simulink model "Robot_leg_1"  (R2017b)
settings: Solver=VariableStepAuto  StartTime=0.0  StopTime=10.0  RelTol=1e-3
model workspace: external: MATLAB File E:\Humanoid\Simscape model\Simscape_model_2\simscape_model\Robot_leg_2_DataFile.m (data not in the file)
values from neighbouring files (symbols this model uses):
  m = 0    [Trajectory_generation.m]    (also in Trajectory_generation_initial.m; final_gait.m)
  smiData =     [matlab_workspace.mat]
undefined symbols (not defined in the file or in its folder): X, Y, Z
libraries: sm_lib x64, simulink x61, nesl_utility x13
(part 1 of 2)
settings Model: Creator=Workstation-1  LastModifiedBy=Workstation-1
settings SolverCC: AlgebraicLoopSolver=LineSearch
settings DiagnosticsConfigSet: SimMechanicsRigidlyBoundBlock=none

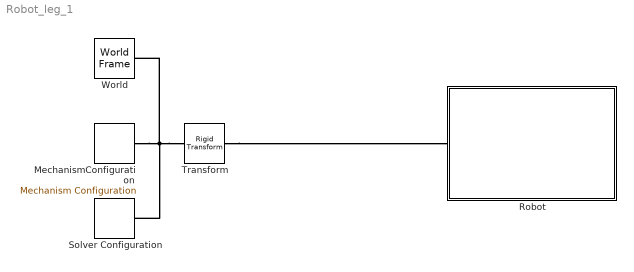
== system Robot_leg_1 ==
  MechanismConfiguration : sm_lib/Utilities/Mechanism Configuration  UniformGravity=Constant  GravityVector=[0 0 -9.80665]  GravityUnits=m/s^2  LinearizationDelta=0.001
  Robot : Subsystem
  Solver Configuration : nesl_utility/Solver Configuration  PhysicalDomain=network_engine_domain  SubClassName=solver  LeftPortType=input  RightPortType=generic  Accelerate=off  Tones=[]  Harmonics=[]  SimulateNoise=off  Profile=off  UseLocalSampling=off  EnableSwitchedLinearOptims=on  FrequencyDomain=off  UseCCode=off  RelTol=0.001  AbsTol=1e-06  MinStep=1e-09  ToWorkspace=off  RevertToSquareIcSolve=off  NumHomotopyIterations=100  PhasorMode=off  PhasorModeNumHarmonics=1  DoDC=off  ResidualTolerance=1e-09  UseLocalSolver=off  LocalSolverChoice=NE_BACKWARD_EULER_ADVANCER  LocalSolverSampleTime=0.001  DoFixedCost=off  MaxNonlinIter=3  MaxModeIter=2  LinearAlgebra=Sparse  DelaysMemoryBudget=1024  AutomaticFiltering=on  FilteringTimeConstant=0.001
  Transform : sm_lib/Frames and Transforms/Rigid Transform  TranslationMethod=Cartesian  TranslationStandardOffset=0  TranslationLengthUnit=mm  TranslationStandardAxis=+Z  TranslationCartesianOffset=smiData.RigidTransform(22).translation  TranslationROffset=0  TranslationROffsetUnits=m  TranslationZOffset=0  TranslationZOffsetUnits=m  TranslationThetaOffset=0  TranslationThetaOffsetUnits=deg  RotationMethod=ArbitraryAxis  RotationAngleUnits=rad  RotationStandardAxis=+Z  RotationAngle=smiData.RigidTransform(22).angle  RotationArbitraryAxis=smiData.RigidTransform(22).axis  FollAlignAxisA=+X  BaseAlignAxisA=+Y  FollAlignAxisB=+Y  BaseAlignAxisB=+Z  RotationSequenceAxes=FollowerAxes  RotationSequence=XYX  RotationSequenceAngles=[0 0 0]  RotationSequenceAnglesUnits=deg  RotationMatrix=[1 0 0; 0 1 0; 0 0 1]
  World : sm_lib/Frames and Transforms/World Frame
  connections:
  Transform/LConn1 -- Solver Configuration/RConn1 -- MechanismConfiguration/RConn1 -- World/RConn1
  Transform/RConn1 -- Robot/RConn1

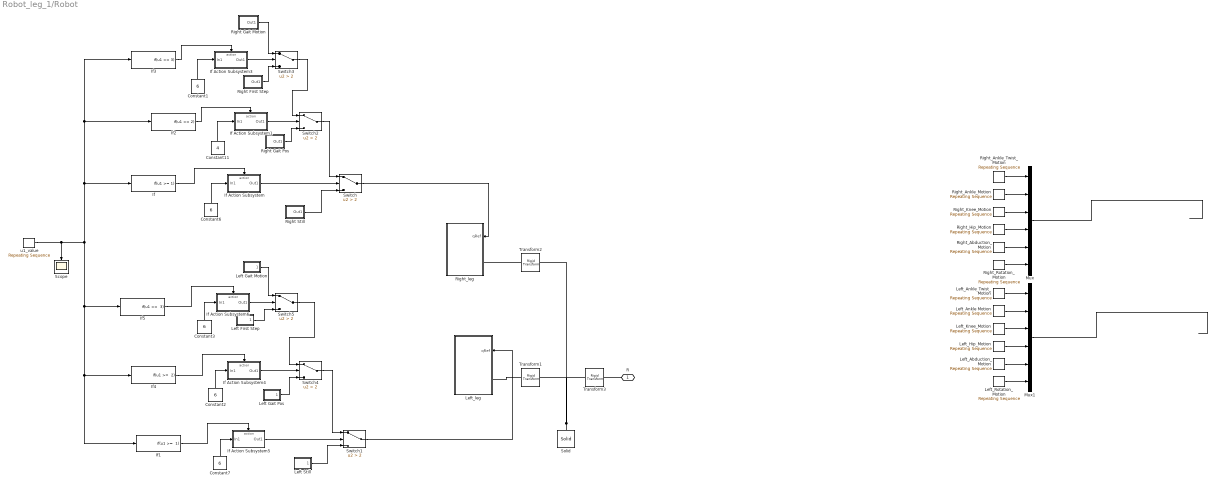
== system Robot_leg_1/Robot ==
  Constant{1..3,6..7} (5 alike) : Constant  Value=6
  Constant11 : Constant  Value=4
  If : If  IfExpression=u1 >= 1  ShowElse=off
  If Action Subsystem : Subsystem  TreatAsAtomicUnit=on
  If Action Subsystem1 : Subsystem  TreatAsAtomicUnit=on
  If Action Subsystem3 : Subsystem  TreatAsAtomicUnit=on
  If Action Subsystem4 : Subsystem  TreatAsAtomicUnit=on
  If Action Subsystem5 : Subsystem  TreatAsAtomicUnit=on
  If Action Subsystem6 : Subsystem  TreatAsAtomicUnit=on
  If1 : If  IfExpression="u1 >=  1"  ShowElse=off
  If2 : If  IfExpression=u1 >= 2  ShowElse=off
  If3 : If  IfExpression=u1 >= 3  ShowElse=off
  If4 : If  IfExpression="u1 >=  2"  ShowElse=off
  If5 : If  IfExpression="u1 >=  3"  ShowElse=off
  Left First Step : Subsystem
  Left Gait Motion : Subsystem
  Left Gait Pos : Subsystem
  Left Still : Subsystem
  Left_Abduction_Motion : simulink/Sources/Repeating Sequence  rep_seq_t=time  rep_seq_y=left_theta_5
  Left_Ankle Motion : simulink/Sources/Repeating Sequence  rep_seq_t=time  rep_seq_y=left_theta_3
  Left_Ankle_Twist_Motion : simulink/Sources/Repeating Sequence  rep_seq_t=time  rep_seq_y=left_theta_4
  Left_Hip_Motion : simulink/Sources/Repeating Sequence  rep_seq_t=time  rep_seq_y=left_theta_1
  Left_Knee_Motion : simulink/Sources/Repeating Sequence  rep_seq_t=time  rep_seq_y=left_theta_2
  Left_Rotation_Motion : simulink/Sources/Repeating Sequence  rep_seq_t=time  rep_seq_y=left_theta_6
  Left_leg : Subsystem
  Mux : Mux  Inputs=6
  Mux1 : Mux  Inputs=6
  Right First Step : Subsystem
  Right Gait Motion : Subsystem
  Right Gait Pos : Subsystem
  Right Still : Subsystem
  Right_Abduction_Motion : simulink/Sources/Repeating Sequence  rep_seq_t=time  rep_seq_y=right_theta_5
  Right_Ankle_Motion : simulink/Sources/Repeating Sequence  rep_seq_t=time  rep_seq_y=right_theta_3
  Right_Ankle_Twist_Motion : simulink/Sources/Repeating Sequence  rep_seq_t=time  rep_seq_y=right_theta_4
  Right_Hip_Motion : simulink/Sources/Repeating Sequence  rep_seq_t=time  rep_seq_y=right_theta_1
  Right_Knee_Motion : simulink/Sources/Repeating Sequence  rep_seq_t=time  rep_seq_y=right_theta_2
  Right_Rotation_Motion : simulink/Sources/Repeating Sequence  rep_seq_t=time  rep_seq_y=right_theta_6
  Right_leg : Subsystem
  Scope : Scope
  Solid : sm_lib/Body Elements/Solid  InertiaType=Custom  Mass=smiData.Solid(13).mass  MassUnits=kg  CenterOfMass=smiData.Solid(13).CoM  CenterOfMassUnits=mm  MomentsOfInertia=smiData.Solid(13).MoI  MomentsOfInertiaUnits=kg*mm^2  ProductsOfInertia=smiData.Solid(13).PoI  ProductsOfInertiaUnits=kg*mm^2  DensityBased=on  Density=1000  DensityUnits=kg/m^3  DoExposeReferenceFrame=on  SerializedFrames=<Frames/>  GraphicType=FromGeometry  MarkerShape=Sphere  MarkerSize=10  GraphicVisPropType=SimpleVisualProperties  GraphicDiffuseColor=smiData.Solid(13).color  GraphicSpecularColor=[0.5 0.5 0.5 1.0]  GraphicAmbientColor=[0.15 0.15 0.15 1.0]  GraphicEmissiveColor=[0.0 0.0 0.0 1.0]  GraphicShininess=75  GraphicOpacity=smiData.Solid(13).opacity  GeometryShape=FromFile  RectangleSize=[1 1]  RectangleSizeUnits=m  BrickDimensions=[1 1 1]  BrickDimensionUnits=m  CylinderRadius=1  CylinderRadiusUnits=m  CylinderLength=1  CylinderLengthUnits=m  SphereRadius=1  SphereRadiusUnits=m  EllipsoidRadii=[1 1 1]  EllipsoidRadiiUnits=m  ExtrusionCrossSection=[1 1; -1 1; -1 -1; 1 -1]  ExtrusionCrossSectionUnits=m  ExtrusionLength=1  ExtrusionLengthUnits=m  PolygonNumSides=3  PolygonOuterRadius=1  PolygonOuterRadiusUnits=m  ExtGeomFileType=STEP  ExtGeomFileName=Torso_Default_sldprt.STEP  ExtGeomFileUnits=m  RevolutionCrossSection=[1 1; 1 -1; 2 -1; 2 1]  RevolutionCrossSectionUnits=m  RevolutionExtent=Full  RevolutionAngle=180  RevolutionAngleUnits=deg
  Switch{,1..5} (6 alike) : Switch  Criteria=u2 > Threshold  Threshold=2
  Transform1 : sm_lib/Frames and Transforms/Rigid Transform  TranslationMethod=Cartesian  TranslationStandardOffset=0  TranslationLengthUnit=mm  TranslationStandardAxis=+Z  TranslationCartesianOffset=smiData.RigidTransform(17).translation  TranslationROffset=0  TranslationROffsetUnits=m  TranslationZOffset=0  TranslationZOffsetUnits=m  TranslationThetaOffset=0  TranslationThetaOffsetUnits=deg  RotationMethod=ArbitraryAxis  RotationAngleUnits=rad  RotationStandardAxis=+Z  RotationAngle=smiData.RigidTransform(17).angle  RotationArbitraryAxis=smiData.RigidTransform(17).axis  FollAlignAxisA=+X  BaseAlignAxisA=+Y  FollAlignAxisB=+Y  BaseAlignAxisB=+Z  RotationSequenceAxes=FollowerAxes  RotationSequence=XYX  RotationSequenceAngles=[0 0 0]  RotationSequenceAnglesUnits=deg  RotationMatrix=[1 0 0; 0 1 0; 0 0 1]
  Transform2 : sm_lib/Frames and Transforms/Rigid Transform  TranslationMethod=Cartesian  TranslationStandardOffset=0  TranslationLengthUnit=mm  TranslationStandardAxis=+Z  TranslationCartesianOffset=smiData.RigidTransform(19).translation  TranslationROffset=0  TranslationROffsetUnits=m  TranslationZOffset=0  TranslationZOffsetUnits=m  TranslationThetaOffset=0  TranslationThetaOffsetUnits=deg  RotationMethod=ArbitraryAxis  RotationAngleUnits=rad  RotationStandardAxis=+Z  RotationAngle=smiData.RigidTransform(19).angle  RotationArbitraryAxis=smiData.RigidTransform(19).axis  FollAlignAxisA=+X  BaseAlignAxisA=+Y  FollAlignAxisB=+Y  BaseAlignAxisB=+Z  RotationSequenceAxes=FollowerAxes  RotationSequence=XYX  RotationSequenceAngles=[0 0 0]  RotationSequenceAnglesUnits=deg  RotationMatrix=[1 0 0; 0 1 0; 0 0 1]
  Transform3 : sm_lib/Frames and Transforms/Rigid Transform  TranslationMethod=Cartesian  TranslationStandardOffset=0  TranslationLengthUnit=mm  TranslationStandardAxis=+Z  TranslationCartesianOffset=smiData.RigidTransform(21).translation  TranslationROffset=0  TranslationROffsetUnits=m  TranslationZOffset=0  TranslationZOffsetUnits=m  TranslationThetaOffset=0  TranslationThetaOffsetUnits=deg  RotationMethod=ArbitraryAxis  RotationAngleUnits=rad  RotationStandardAxis=+Z  RotationAngle=smiData.RigidTransform(21).angle  RotationArbitraryAxis=smiData.RigidTransform(21).axis  FollAlignAxisA=+X  BaseAlignAxisA=+Y  FollAlignAxisB=+Y  BaseAlignAxisB=+Z  RotationSequenceAxes=FollowerAxes  RotationSequence=XYX  RotationSequenceAngles=[0 0 0]  RotationSequenceAnglesUnits=deg  RotationMatrix=[1 0 0; 0 1 0; 0 0 1]
  "u1_value " : simulink/Sources/Repeating Sequence  rep_seq_t=total_time  rep_seq_y=u1
  R : PMIOPort  Port=1  Side=Right
  wires:
  If Action Subsystem1/1(Out1) -> Switch2/2
  If3/1 -> If Action Subsystem3/Action
  Constant3/1 -> If Action Subsystem6/1(In1)
  If5/1 -> If Action Subsystem6/Action
  Switch4/1 -> Switch1/1
  If Action Subsystem3/1(Out1) -> Switch3/2
  If4/1 -> If Action Subsystem4/Action
  Constant2/1 -> If Action Subsystem4/1(In1)
  If Action Subsystem5/1(Out1) -> Switch1/2
  If Action Subsystem6/1(Out1) -> Switch5/2
  Switch3/1 -> Switch2/1
  If Action Subsystem/1(Out1) -> Switch/2
  Constant7/1 -> If Action Subsystem5/1(In1)
  If/1 -> If Action Subsystem/Action
  If Action Subsystem4/1(Out1) -> Switch4/2
  Constant1/1 -> If Action Subsystem3/1(In1)
  If2/1 -> If Action Subsystem1/Action
  Switch5/1 -> Switch4/1
  Left Gait Pos/1(Out1) -> Switch4/3
  Constant6/1 -> If Action Subsystem/1(In1)
  Switch2/1 -> Switch/1
  If1/1 -> If Action Subsystem5/Action
  Constant11/1 -> If Action Subsystem1/1(In1)
  Left_Rotation_Motion/1 -> Mux1/6
  Left_Knee_Motion/1 -> Mux1/3
  Left_Hip_Motion/1 -> Mux1/4
  Left_Ankle_Twist_Motion/1 -> Mux1/1
  Right_Rotation_Motion/1 -> Mux/6
  Mux1/1 -> ?
  Right_Ankle_Motion/1 -> Mux/2
  Mux/1 -> ?
  Left_Abduction_Motion/1 -> Mux1/5
  Right_Abduction_Motion/1 -> Mux/5
  Right_Knee_Motion/1 -> Mux/3
  Right_Hip_Motion/1 -> Mux/4
  Left_Ankle Motion/1 -> Mux1/2
  Right_Ankle_Twist_Motion/1 -> Mux/1
  Switch/1 -> Right_leg/1(qRef)
  Switch1/1 -> Left_leg/1(qRef)
  Left First Step/1(Out1) -> Switch5/3
  Right Gait Pos/1(Out1) -> Switch2/3
  "u1_value "/1 -> Scope/1, If5/1, If4/1, If1/1, If2/1, If3/1, If/1
  Right First Step/1(Out1) -> Switch3/3
  Right Gait Motion/1(Out1) -> Switch3/1
  Right Still/1(Out1) -> Switch/3
  Left Gait Motion/1(Out1) -> Switch5/1
  Left Still/1(Out1) -> Switch1/3
  connections:
  Solid/RConn1 -- Transform2/LConn1 -- Transform1/LConn1 -- Transform3/LConn1
  R/RConn1 -- Transform3/RConn1
  Transform2/RConn1 -- Right_leg/LConn1
  Transform1/RConn1 -- Left_leg/LConn1

== system Robot_leg_1/Robot/If Action Subsystem ==
  In1 : Inport
  Action Port : ActionPort  ActionType=then
  Out1 : Outport
  wires:
  In1/1 -> Out1/1

== system Robot_leg_1/Robot/If Action Subsystem1 ==
  In1 : Inport
  Action Port : ActionPort  ActionType=then
  Out1 : Outport
  wires:
  In1/1 -> Out1/1

== system Robot_leg_1/Robot/If Action Subsystem3 ==
  In1 : Inport
  Action Port : ActionPort  ActionType=then
  Out1 : Outport
  wires:
  In1/1 -> Out1/1

== system Robot_leg_1/Robot/If Action Subsystem4 ==
  In1 : Inport
  Action Port : ActionPort  ActionType=then
  Out1 : Outport
  wires:
  In1/1 -> Out1/1

== system Robot_leg_1/Robot/If Action Subsystem5 ==
  In1 : Inport
  Action Port : ActionPort  ActionType=then
  Out1 : Outport
  wires:
  In1/1 -> Out1/1

== system Robot_leg_1/Robot/If Action Subsystem6 ==
  In1 : Inport
  Action Port : ActionPort  ActionType=then
  Out1 : Outport
  wires:
  In1/1 -> Out1/1

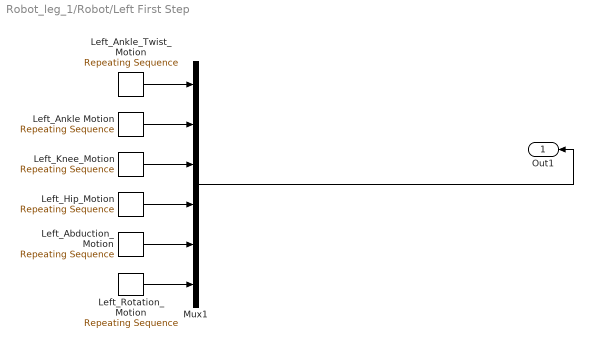
== system Robot_leg_1/Robot/Left First Step ==
  Left_Abduction_Motion : simulink/Sources/Repeating Sequence  rep_seq_t=time  rep_seq_y=left_theta_first_5
  Left_Ankle Motion : simulink/Sources/Repeating Sequence  rep_seq_t=time_first  rep_seq_y=left_theta_first_3
  Left_Ankle_Twist_Motion : simulink/Sources/Repeating Sequence  rep_seq_t=time  rep_seq_y=left_theta_first_4
  Left_Hip_Motion : simulink/Sources/Repeating Sequence  rep_seq_t=time_first  rep_seq_y=left_theta_first_1
  Left_Knee_Motion : simulink/Sources/Repeating Sequence  rep_seq_t=time_first  rep_seq_y=left_theta_first_2
  Left_Rotation_Motion : simulink/Sources/Repeating Sequence  rep_seq_t=time_first  rep_seq_y=left_theta_first_6
  Mux1 : Mux  Inputs=6
  Out1 : Outport
  wires:
  Left_Knee_Motion/1 -> Mux1/3
  Left_Rotation_Motion/1 -> Mux1/6
  Left_Hip_Motion/1 -> Mux1/4
  Left_Abduction_Motion/1 -> Mux1/5
  Left_Ankle_Twist_Motion/1 -> Mux1/1
  Left_Ankle Motion/1 -> Mux1/2
  Mux1/1 -> Out1/1

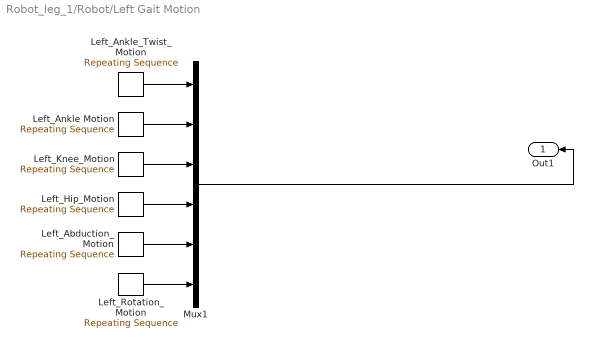
== system Robot_leg_1/Robot/Left Gait Motion ==
  Left_Abduction_Motion : simulink/Sources/Repeating Sequence  rep_seq_t=time  rep_seq_y=left_theta_5
  Left_Ankle Motion : simulink/Sources/Repeating Sequence  rep_seq_t=time  rep_seq_y=left_theta_3
  Left_Ankle_Twist_Motion : simulink/Sources/Repeating Sequence  rep_seq_t=time  rep_seq_y=left_theta_4
  Left_Hip_Motion : simulink/Sources/Repeating Sequence  rep_seq_t=time  rep_seq_y=left_theta_1
  Left_Knee_Motion : simulink/Sources/Repeating Sequence  rep_seq_t=time  rep_seq_y=left_theta_2
  Left_Rotation_Motion : simulink/Sources/Repeating Sequence  rep_seq_t=time  rep_seq_y=left_theta_6
  Mux1 : Mux  Inputs=6
  Out1 : Outport
  wires:
  Left_Knee_Motion/1 -> Mux1/3
  Left_Rotation_Motion/1 -> Mux1/6
  Left_Hip_Motion/1 -> Mux1/4
  Left_Abduction_Motion/1 -> Mux1/5
  Left_Ankle_Twist_Motion/1 -> Mux1/1
  Left_Ankle Motion/1 -> Mux1/2
  Mux1/1 -> Out1/1

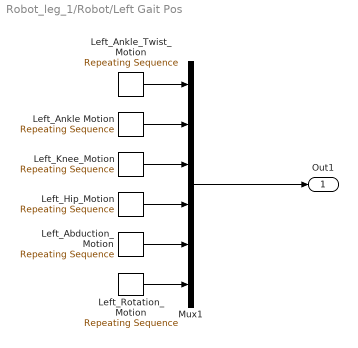
== system Robot_leg_1/Robot/Left Gait Pos ==
  Left_Abduction_Motion : simulink/Sources/Repeating Sequence  rep_seq_t=time  rep_seq_y=left_theta_pos_5
  Left_Ankle Motion : simulink/Sources/Repeating Sequence  rep_seq_t=time  rep_seq_y=left_theta_pos_3
  Left_Ankle_Twist_Motion : simulink/Sources/Repeating Sequence  rep_seq_t=time  rep_seq_y=left_theta_pos_4
  Left_Hip_Motion : simulink/Sources/Repeating Sequence  rep_seq_t=time  rep_seq_y=left_theta_pos_1
  Left_Knee_Motion : simulink/Sources/Repeating Sequence  rep_seq_t=time  rep_seq_y=left_theta_pos_2
  Left_Rotation_Motion : simulink/Sources/Repeating Sequence  rep_seq_t=time  rep_seq_y=left_theta_pos_6
  Mux1 : Mux  Inputs=6
  Out1 : Outport
  wires:
  Mux1/1 -> Out1/1
  Left_Ankle Motion/1 -> Mux1/2
  Left_Ankle_Twist_Motion/1 -> Mux1/1
  Left_Abduction_Motion/1 -> Mux1/5
  Left_Hip_Motion/1 -> Mux1/4
  Left_Rotation_Motion/1 -> Mux1/6
  Left_Knee_Motion/1 -> Mux1/3

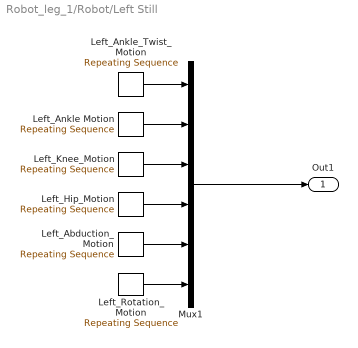
== system Robot_leg_1/Robot/Left Still ==
  Left_Abduction_Motion : simulink/Sources/Repeating Sequence  rep_seq_t=time  rep_seq_y=left_theta_init_5
  Left_Ankle Motion : simulink/Sources/Repeating Sequence  rep_seq_t=time  rep_seq_y=left_theta_init_3
  Left_Ankle_Twist_Motion : simulink/Sources/Repeating Sequence  rep_seq_t=time  rep_seq_y=left_theta_init_4
  Left_Hip_Motion : simulink/Sources/Repeating Sequence  rep_seq_t=time  rep_seq_y=left_theta_init_1
  Left_Knee_Motion : simulink/Sources/Repeating Sequence  rep_seq_t=time  rep_seq_y=left_theta_init_2
  Left_Rotation_Motion : simulink/Sources/Repeating Sequence  rep_seq_t=time  rep_seq_y=left_theta_init_6
  Mux1 : Mux  Inputs=6
  Out1 : Outport
  wires:
  Mux1/1 -> Out1/1
  Left_Ankle Motion/1 -> Mux1/2
  Left_Ankle_Twist_Motion/1 -> Mux1/1
  Left_Abduction_Motion/1 -> Mux1/5
  Left_Hip_Motion/1 -> Mux1/4
  Left_Rotation_Motion/1 -> Mux1/6
  Left_Knee_Motion/1 -> Mux1/3

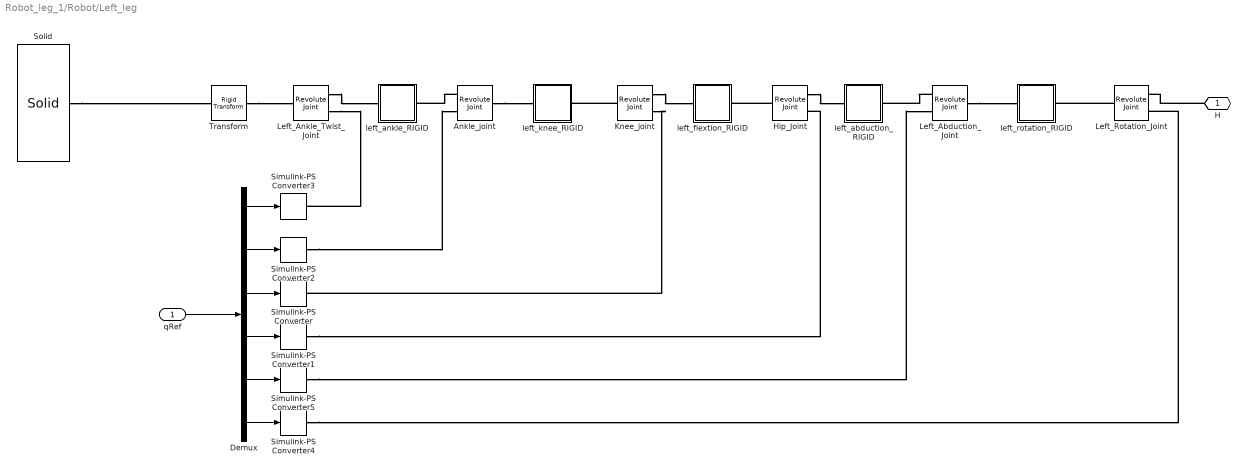
== system Robot_leg_1/Robot/Left_leg ==
  qRef : Inport
  Ankle_joint : sm_lib/Joints/Revolute Joint  SenseConstraintForce=off  SenseConstraintForceX=off  SenseConstraintForceY=off  SenseConstraintForceZ=off  SenseConstraintTorque=off  SenseConstraintTorqueX=off  SenseConstraintTorqueY=off  SenseConstraintTorqueZ=off  SenseTotalForce=off  SenseTotalForceX=off  SenseTotalForceY=off  SenseTotalForceZ=off  SenseTotalTorque=off  SenseTotalTorqueX=off  SenseTotalTorqueY=off  SenseTotalTorqueZ=off  CompositeWrenchDir=FollowerOnBase  CompositeWrenchFrame=BaseFrame  EquilibriumPosition=0  EquilibriumPositionUnits=rad  SpringStiffness=0  SpringStiffnessUnits=N*m/rad  DampingCoefficient=0  DampingCoefficientUnits=N*m/(rad/s)  TorqueActuationMode=ComputedTorque  MotionActuationMode=InputMotion  SensePosition=off  SenseVelocity=off  SenseAcceleration=off  SenseTorqueForce=off  PositionTargetSpecify=on  PositionTargetPriority=Low  PositionTargetValue=smiData.RevoluteJoint(7).Rz.Pos  PositionTargetValueUnits=deg  VelocityTargetSpecify=off  VelocityTargetPriority=High  VelocityTargetValue=0  VelocityTargetValueUnits=deg/s
  Demux : Demux  Outputs=6
  Hip_Joint : sm_lib/Joints/Revolute Joint  SenseConstraintForce=off  SenseConstraintForceX=off  SenseConstraintForceY=off  SenseConstraintForceZ=off  SenseConstraintTorque=off  SenseConstraintTorqueX=off  SenseConstraintTorqueY=off  SenseConstraintTorqueZ=off  SenseTotalForce=off  SenseTotalForceX=off  SenseTotalForceY=off  SenseTotalForceZ=off  SenseTotalTorque=off  SenseTotalTorqueX=off  SenseTotalTorqueY=off  SenseTotalTorqueZ=off  CompositeWrenchDir=FollowerOnBase  CompositeWrenchFrame=BaseFrame  EquilibriumPosition=0  EquilibriumPositionUnits=rad  SpringStiffness=0  SpringStiffnessUnits=N*m/rad  DampingCoefficient=0  DampingCoefficientUnits=N*m/(rad/s)  TorqueActuationMode=ComputedTorque  MotionActuationMode=InputMotion  SensePosition=off  SenseVelocity=off  SenseAcceleration=off  SenseTorqueForce=off  PositionTargetSpecify=on  PositionTargetPriority=Low  PositionTargetValue=smiData.RevoluteJoint(12).Rz.Pos  PositionTargetValueUnits=deg  VelocityTargetSpecify=off  VelocityTargetPriority=High  VelocityTargetValue=0  VelocityTargetValueUnits=deg/s
  Knee_joint : sm_lib/Joints/Revolute Joint  SenseConstraintForce=off  SenseConstraintForceX=off  SenseConstraintForceY=off  SenseConstraintForceZ=off  SenseConstraintTorque=off  SenseConstraintTorqueX=off  SenseConstraintTorqueY=off  SenseConstraintTorqueZ=off  SenseTotalForce=off  SenseTotalForceX=off  SenseTotalForceY=off  SenseTotalForceZ=off  SenseTotalTorque=off  SenseTotalTorqueX=off  SenseTotalTorqueY=off  SenseTotalTorqueZ=off  CompositeWrenchDir=FollowerOnBase  CompositeWrenchFrame=BaseFrame  EquilibriumPosition=0  EquilibriumPositionUnits=rad  SpringStiffness=0  SpringStiffnessUnits=N*m/rad  DampingCoefficient=0  DampingCoefficientUnits=N*m/(rad/s)  TorqueActuationMode=ComputedTorque  MotionActuationMode=InputMotion  SensePosition=off  SenseVelocity=off  SenseAcceleration=off  SenseTorqueForce=off  PositionTargetSpecify=on  PositionTargetPriority=Low  PositionTargetValue=smiData.RevoluteJoint(11).Rz.Pos  PositionTargetValueUnits=deg  VelocityTargetSpecify=off  VelocityTargetPriority=High  VelocityTargetValue=0  VelocityTargetValueUnits=deg/s
  Left_Abduction_Joint : sm_lib/Joints/Revolute Joint  SenseConstraintForce=off  SenseConstraintForceX=off  SenseConstraintForceY=off  SenseConstraintForceZ=off  SenseConstraintTorque=off  SenseConstraintTorqueX=off  SenseConstraintTorqueY=off  SenseConstraintTorqueZ=off  SenseTotalForce=off  SenseTotalForceX=off  SenseTotalForceY=off  SenseTotalForceZ=off  SenseTotalTorque=off  SenseTotalTorqueX=off  SenseTotalTorqueY=off  SenseTotalTorqueZ=off  CompositeWrenchDir=FollowerOnBase  CompositeWrenchFrame=BaseFrame  EquilibriumPosition=0  EquilibriumPositionUnits=rad  SpringStiffness=0  SpringStiffnessUnits=N*m/rad  DampingCoefficient=0  DampingCoefficientUnits=N*m/(rad/s)  TorqueActuationMode=ComputedTorque  MotionActuationMode=InputMotion  SensePosition=off  SenseVelocity=off  SenseAcceleration=off  SenseTorqueForce=off  PositionTargetSpecify=on  PositionTargetPriority=Low  PositionTargetValue=smiData.RevoluteJoint(4).Rz.Pos  PositionTargetValueUnits=deg  VelocityTargetSpecify=off  VelocityTargetPriority=High  VelocityTargetValue=0  VelocityTargetValueUnits=deg/s
  Left_Ankle_Twist_Joint : sm_lib/Joints/Revolute Joint  SenseConstraintForce=off  SenseConstraintForceX=off  SenseConstraintForceY=off  SenseConstraintForceZ=off  SenseConstraintTorque=off  SenseConstraintTorqueX=off  SenseConstraintTorqueY=off  SenseConstraintTorqueZ=off  SenseTotalForce=off  SenseTotalForceX=off  SenseTotalForceY=off  SenseTotalForceZ=off  SenseTotalTorque=off  SenseTotalTorqueX=off  SenseTotalTorqueY=off  SenseTotalTorqueZ=off  CompositeWrenchDir=FollowerOnBase  CompositeWrenchFrame=BaseFrame  EquilibriumPosition=0  EquilibriumPositionUnits=rad  SpringStiffness=0  SpringStiffnessUnits=N*m/rad  DampingCoefficient=0  DampingCoefficientUnits=N*m/(rad/s)  TorqueActuationMode=ComputedTorque  MotionActuationMode=InputMotion  SensePosition=off  SenseVelocity=off  SenseAcceleration=off  SenseTorqueForce=off  PositionTargetSpecify=on  PositionTargetPriority=Low  PositionTargetValue=smiData.RevoluteJoint(6).Rz.Pos  PositionTargetValueUnits=deg  VelocityTargetSpecify=off  VelocityTargetPriority=High  VelocityTargetValue=0  VelocityTargetValueUnits=deg/s
  Left_Rotation_Joint : sm_lib/Joints/Revolute Joint  SenseConstraintForce=off  SenseConstraintForceX=off  SenseConstraintForceY=off  SenseConstraintForceZ=off  SenseConstraintTorque=off  SenseConstraintTorqueX=off  SenseConstraintTorqueY=off  SenseConstraintTorqueZ=off  SenseTotalForce=off  SenseTotalForceX=off  SenseTotalForceY=off  SenseTotalForceZ=off  SenseTotalTorque=off  SenseTotalTorqueX=off  SenseTotalTorqueY=off  SenseTotalTorqueZ=off  CompositeWrenchDir=FollowerOnBase  CompositeWrenchFrame=BaseFrame  EquilibriumPosition=0  EquilibriumPositionUnits=rad  SpringStiffness=0  SpringStiffnessUnits=N*m/rad  DampingCoefficient=0  DampingCoefficientUnits=N*m/(rad/s)  TorqueActuationMode=ComputedTorque  MotionActuationMode=InputMotion  SensePosition=off  SenseVelocity=off  SenseAcceleration=off  SenseTorqueForce=off  PositionTargetSpecify=on  PositionTargetPriority=Low  PositionTargetValue=smiData.RevoluteJoint(9).Rz.Pos  PositionTargetValueUnits=deg  VelocityTargetSpecify=off  VelocityTargetPriority=High  VelocityTargetValue=0  VelocityTargetValueUnits=deg/s
  Simulink-PS Converter{,1..5} (6 alike) : nesl_utility/Simulink-PS Converter  PhysicalDomain=network_engine_domain  SubClassName=ps_input  LeftPortType=input  RightPortType=output  PseudoPeriodic=off  Frequencies=[]  NoiseDistribution=none  NoiseParameters=[]  Unit=rad  AffineConversion=off  FilteringAndDerivatives=filter  SimscapeFilterOrder=2  InputFilterTimeConstant=motion_time_constant  UdotUserProvided=1
  Solid : sm_lib/Body Elements/Solid  InertiaType=Custom  Mass=smiData.Solid(10).mass  MassUnits=kg  CenterOfMass=smiData.Solid(10).CoM  CenterOfMassUnits=mm  MomentsOfInertia=smiData.Solid(10).MoI  MomentsOfInertiaUnits=kg*mm^2  ProductsOfInertia=smiData.Solid(10).PoI  ProductsOfInertiaUnits=kg*mm^2  DensityBased=on  Density=1000  DensityUnits=kg/m^3  DoExposeReferenceFrame=on  SerializedFrames=<Frames/>  GraphicType=FromGeometry  MarkerShape=Sphere  MarkerSize=10  GraphicVisPropType=SimpleVisualProperties  GraphicDiffuseColor=smiData.Solid(10).color  GraphicSpecularColor=[0.5 0.5 0.5 1.0]  GraphicAmbientColor=[0.15 0.15 0.15 1.0]  GraphicEmissiveColor=[0.0 0.0 0.0 1.0]  GraphicShininess=75  GraphicOpacity=smiData.Solid(10).opacity  GeometryShape=FromFile  RectangleSize=[1 1]  RectangleSizeUnits=m  BrickDimensions=[1 1 1]  BrickDimensionUnits=m  CylinderRadius=1  CylinderRadiusUnits=m  CylinderLength=1  CylinderLengthUnits=m  SphereRadius=1  SphereRadiusUnits=m  EllipsoidRadii=[1 1 1]  EllipsoidRadiiUnits=m  ExtrusionCrossSection=[1 1; -1 1; -1 -1; 1 -1]  ExtrusionCrossSectionUnits=m  ExtrusionLength=1  ExtrusionLengthUnits=m  PolygonNumSides=3  PolygonOuterRadius=1  PolygonOuterRadiusUnits=m  ExtGeomFileType=STEP  ExtGeomFileName=left_ankle_twist_part_Default_sldprt.STEP  ExtGeomFileUnits=m  RevolutionCrossSection=[1 1; 1 -1; 2 -1; 2 1]  RevolutionCrossSectionUnits=m  RevolutionExtent=Full  RevolutionAngle=180  RevolutionAngleUnits=deg
  Transform : sm_lib/Frames and Transforms/Rigid Transform  TranslationMethod=Cartesian  TranslationStandardOffset=0  TranslationLengthUnit=mm  TranslationStandardAxis=+Z  TranslationCartesianOffset=smiData.RigidTransform(12).translation  TranslationROffset=0  TranslationROffsetUnits=m  TranslationZOffset=0  TranslationZOffsetUnits=m  TranslationThetaOffset=0  TranslationThetaOffsetUnits=deg  RotationMethod=ArbitraryAxis  RotationAngleUnits=rad  RotationStandardAxis=+Z  RotationAngle=smiData.RigidTransform(12).angle  RotationArbitraryAxis=smiData.RigidTransform(12).axis  FollAlignAxisA=+X  BaseAlignAxisA=+Y  FollAlignAxisB=+Y  BaseAlignAxisB=+Z  RotationSequenceAxes=FollowerAxes  RotationSequence=XYX  RotationSequenceAngles=[0 0 0]  RotationSequenceAnglesUnits=deg  RotationMatrix=[1 0 0; 0 1 0; 0 0 1]
  left_abduction_RIGID : Subsystem
  left_ankle_RIGID : Subsystem
  left_flextion_RIGID : Subsystem
  left_knee_RIGID : Subsystem
  left_rotation_RIGID : Subsystem
  H : PMIOPort  Port=1  Side=Left
  wires:
  Demux/3 -> Simulink-PS Converter/1
  Demux/4 -> Simulink-PS Converter1/1
  Demux/5 -> Simulink-PS Converter5/1
  Demux/6 -> Simulink-PS Converter4/1
  Demux/2 -> Simulink-PS Converter2/1
  Demux/1 -> Simulink-PS Converter3/1
  qRef/1 -> Demux/1
  connections:
  Knee_joint/LConn1 -- left_flextion_RIGID/RConn1
  Ankle_joint/RConn1 -- left_knee_RIGID/LConn1
  Ankle_joint/LConn1 -- left_ankle_RIGID/RConn1
  H/RConn1 -- Left_Rotation_Joint/LConn1
  Left_Ankle_Twist_Joint/LConn1 -- left_ankle_RIGID/LConn1
  Left_Rotation_Joint/RConn1 -- left_rotation_RIGID/RConn1
  Hip_Joint/LConn1 -- left_abduction_RIGID/RConn1
  Knee_joint/RConn1 -- left_knee_RIGID/RConn1
  Left_Abduction_Joint/LConn1 -- left_abduction_RIGID/LConn1
  Hip_Joint/RConn1 -- left_flextion_RIGID/LConn1
  Left_Abduction_Joint/RConn1 -- left_rotation_RIGID/LConn1
  Transform/RConn1 -- Left_Ankle_Twist_Joint/RConn1
  Solid/RConn1 -- Transform/LConn1
  Simulink-PS Converter4/RConn1 -- Left_Rotation_Joint/LConn2
  Simulink-PS Converter5/RConn1 -- Left_Abduction_Joint/LConn2
  Knee_joint/LConn2 -- Simulink-PS Converter/RConn1
  Simulink-PS Converter1/RConn1 -- Hip_Joint/LConn2
  Simulink-PS Converter2/RConn1 -- Ankle_joint/LConn2
  Left_Ankle_Twist_Joint/LConn2 -- Simulink-PS Converter3/RConn1

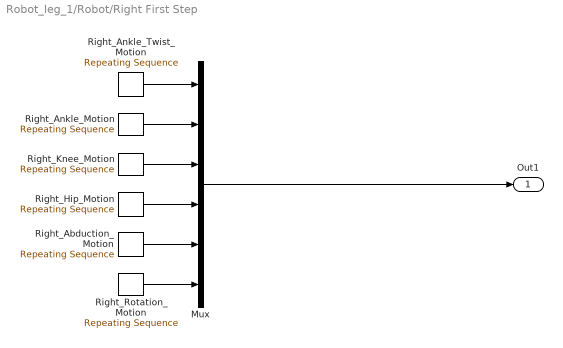
== system Robot_leg_1/Robot/Right First Step ==
  Mux : Mux  Inputs=6
  Right_Abduction_Motion : simulink/Sources/Repeating Sequence  rep_seq_t=time  rep_seq_y=right_theta_first_5
  Right_Ankle_Motion : simulink/Sources/Repeating Sequence  rep_seq_t=time  rep_seq_y=right_theta_first_3
  Right_Ankle_Twist_Motion : simulink/Sources/Repeating Sequence  rep_seq_t=time  rep_seq_y=right_theta_first_4
  Right_Hip_Motion : simulink/Sources/Repeating Sequence  rep_seq_t=time  rep_seq_y=right_theta_first_1
  Right_Knee_Motion : simulink/Sources/Repeating Sequence  rep_seq_t=time  rep_seq_y=right_theta_first_2
  Right_Rotation_Motion : simulink/Sources/Repeating Sequence  rep_seq_t=time_first  rep_seq_y=right_theta_first_6
  Out1 : Outport
  wires:
  Mux/1 -> Out1/1
  Right_Ankle_Motion/1 -> Mux/2
  Right_Ankle_Twist_Motion/1 -> Mux/1
  Right_Knee_Motion/1 -> Mux/3
  Right_Rotation_Motion/1 -> Mux/6
  Right_Abduction_Motion/1 -> Mux/5
  Right_Hip_Motion/1 -> Mux/4

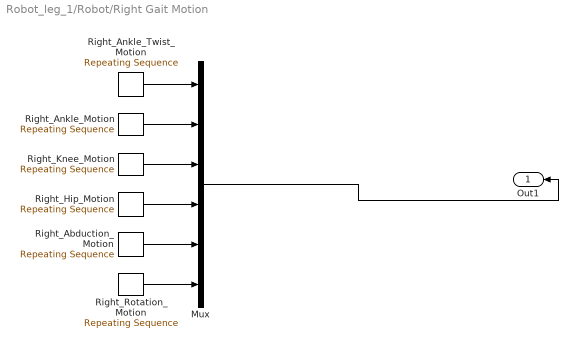
== system Robot_leg_1/Robot/Right Gait Motion ==
  Mux : Mux  Inputs=6
  Right_Abduction_Motion : simulink/Sources/Repeating Sequence  rep_seq_t=time  rep_seq_y=right_theta_5
  Right_Ankle_Motion : simulink/Sources/Repeating Sequence  rep_seq_t=time  rep_seq_y=right_theta_3
  Right_Ankle_Twist_Motion : simulink/Sources/Repeating Sequence  rep_seq_t=time  rep_seq_y=right_theta_4
  Right_Hip_Motion : simulink/Sources/Repeating Sequence  rep_seq_t=time  rep_seq_y=right_theta_1
  Right_Knee_Motion : simulink/Sources/Repeating Sequence  rep_seq_t=time  rep_seq_y=right_theta_2
  Right_Rotation_Motion : simulink/Sources/Repeating Sequence  rep_seq_t=time  rep_seq_y=right_theta_6
  Out1 : Outport
  wires:
  Mux/1 -> Out1/1
  Right_Ankle_Motion/1 -> Mux/2
  Right_Ankle_Twist_Motion/1 -> Mux/1
  Right_Knee_Motion/1 -> Mux/3
  Right_Rotation_Motion/1 -> Mux/6
  Right_Abduction_Motion/1 -> Mux/5
  Right_Hip_Motion/1 -> Mux/4

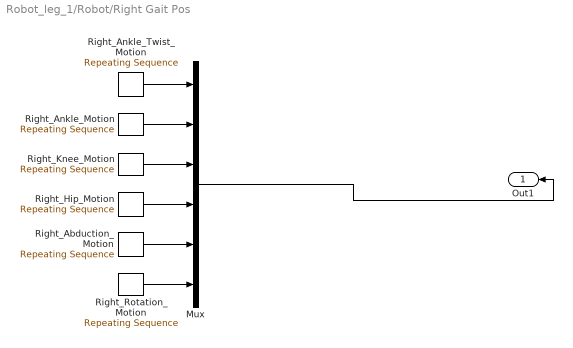
== system Robot_leg_1/Robot/Right Gait Pos ==
  Mux : Mux  Inputs=6
  Right_Abduction_Motion : simulink/Sources/Repeating Sequence  rep_seq_t=time  rep_seq_y=right_theta_pos_5
  Right_Ankle_Motion : simulink/Sources/Repeating Sequence  rep_seq_t=time  rep_seq_y=right_theta_pos_3
  Right_Ankle_Twist_Motion : simulink/Sources/Repeating Sequence  rep_seq_t=time  rep_seq_y=right_theta_pos_4
  Right_Hip_Motion : simulink/Sources/Repeating Sequence  rep_seq_t=time  rep_seq_y=right_theta_pos_1
  Right_Knee_Motion : simulink/Sources/Repeating Sequence  rep_seq_t=time  rep_seq_y=right_theta_pos_2
  Right_Rotation_Motion : simulink/Sources/Repeating Sequence  rep_seq_t=time  rep_seq_y=right_theta_pos_6
  Out1 : Outport
  wires:
  Mux/1 -> Out1/1
  Right_Rotation_Motion/1 -> Mux/6
  Right_Hip_Motion/1 -> Mux/4
  Right_Ankle_Twist_Motion/1 -> Mux/1
  Right_Knee_Motion/1 -> Mux/3
  Right_Abduction_Motion/1 -> Mux/5
  Right_Ankle_Motion/1 -> Mux/2

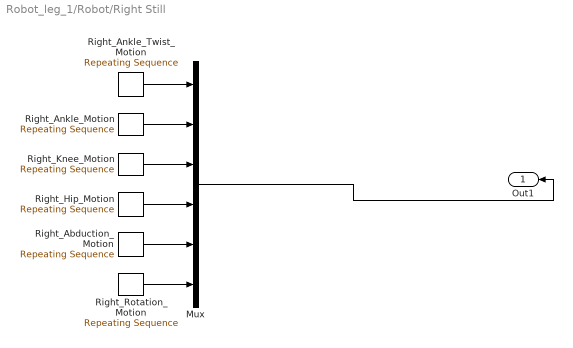
== system Robot_leg_1/Robot/Right Still ==
  Mux : Mux  Inputs=6
  Right_Abduction_Motion : simulink/Sources/Repeating Sequence  rep_seq_t=time  rep_seq_y=right_theta_init_5
  Right_Ankle_Motion : simulink/Sources/Repeating Sequence  rep_seq_t=time  rep_seq_y=right_theta_init_3
  Right_Ankle_Twist_Motion : simulink/Sources/Repeating Sequence  rep_seq_t=time  rep_seq_y=right_theta_init_4
  Right_Hip_Motion : simulink/Sources/Repeating Sequence  rep_seq_t=time  rep_seq_y=right_theta_init_1
  Right_Knee_Motion : simulink/Sources/Repeating Sequence  rep_seq_t=time  rep_seq_y=right_theta_init_2
  Right_Rotation_Motion : simulink/Sources/Repeating Sequence  rep_seq_t=time  rep_seq_y=right_theta_init_6
  Out1 : Outport
  wires:
  Mux/1 -> Out1/1
  Right_Rotation_Motion/1 -> Mux/6
  Right_Hip_Motion/1 -> Mux/4
  Right_Ankle_Twist_Motion/1 -> Mux/1
  Right_Knee_Motion/1 -> Mux/3
  Right_Abduction_Motion/1 -> Mux/5
  Right_Ankle_Motion/1 -> Mux/2

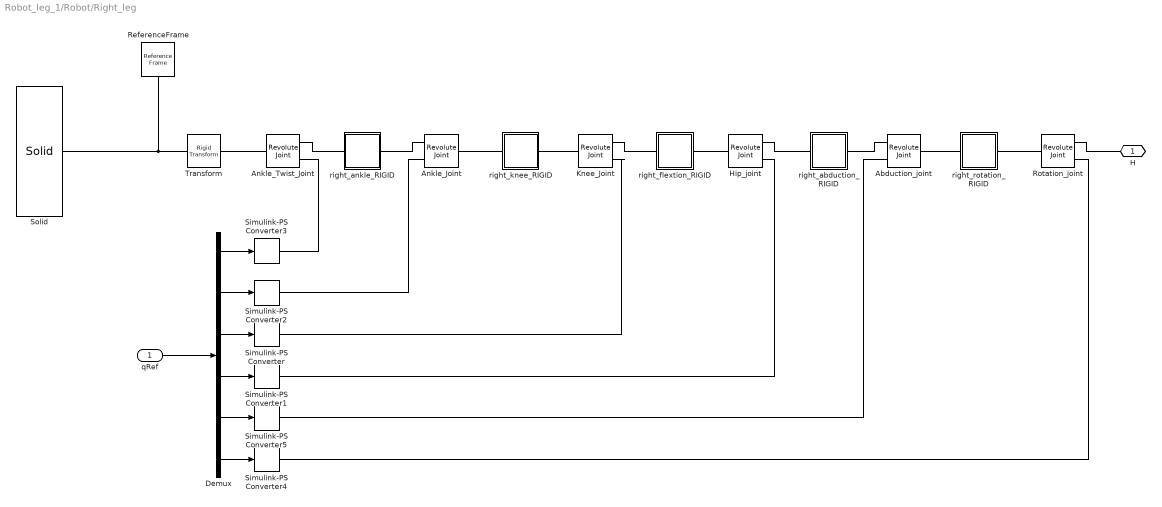
== system Robot_leg_1/Robot/Right_leg ==
  qRef : Inport
  Abduction_joint : sm_lib/Joints/Revolute Joint  SenseConstraintForce=off  SenseConstraintForceX=off  SenseConstraintForceY=off  SenseConstraintForceZ=off  SenseConstraintTorque=off  SenseConstraintTorqueX=off  SenseConstraintTorqueY=off  SenseConstraintTorqueZ=off  SenseTotalForce=off  SenseTotalForceX=off  SenseTotalForceY=off  SenseTotalForceZ=off  SenseTotalTorque=off  SenseTotalTorqueX=off  SenseTotalTorqueY=off  SenseTotalTorqueZ=off  CompositeWrenchDir=FollowerOnBase  CompositeWrenchFrame=BaseFrame  EquilibriumPosition=0  EquilibriumPositionUnits=rad  SpringStiffness=0  SpringStiffnessUnits=N*m/rad  DampingCoefficient=0  DampingCoefficientUnits=N*m/(rad/s)  TorqueActuationMode=ComputedTorque  MotionActuationMode=InputMotion  SensePosition=off  SenseVelocity=off  SenseAcceleration=off  SenseTorqueForce=off  PositionTargetSpecify=on  PositionTargetPriority=Low  PositionTargetValue=smiData.RevoluteJoint(5).Rz.Pos  PositionTargetValueUnits=deg  VelocityTargetSpecify=off  VelocityTargetPriority=High  VelocityTargetValue=0  VelocityTargetValueUnits=deg/s
  Ankle_Joint : sm_lib/Joints/Revolute Joint  SenseConstraintForce=off  SenseConstraintForceX=off  SenseConstraintForceY=off  SenseConstraintForceZ=off  SenseConstraintTorque=off  SenseConstraintTorqueX=off  SenseConstraintTorqueY=off  SenseConstraintTorqueZ=off  SenseTotalForce=off  SenseTotalForceX=off  SenseTotalForceY=off  SenseTotalForceZ=off  SenseTotalTorque=off  SenseTotalTorqueX=off  SenseTotalTorqueY=off  SenseTotalTorqueZ=off  CompositeWrenchDir=FollowerOnBase  CompositeWrenchFrame=BaseFrame  EquilibriumPosition=0  EquilibriumPositionUnits=rad  SpringStiffness=0  SpringStiffnessUnits=N*m/rad  DampingCoefficient=0  DampingCoefficientUnits=N*m/(rad/s)  TorqueActuationMode=ComputedTorque  MotionActuationMode=InputMotion  SensePosition=off  SenseVelocity=off  SenseAcceleration=off  SenseTorqueForce=off  PositionTargetSpecify=on  PositionTargetPriority=Low  PositionTargetValue=smiData.RevoluteJoint(3).Rz.Pos  PositionTargetValueUnits=deg  VelocityTargetSpecify=off  VelocityTargetPriority=High  VelocityTargetValue=0  VelocityTargetValueUnits=deg/s
  Ankle_Twist_Joint : sm_lib/Joints/Revolute Joint  SenseConstraintForce=off  SenseConstraintForceX=off  SenseConstraintForceY=off  SenseConstraintForceZ=off  SenseConstraintTorque=off  SenseConstraintTorqueX=off  SenseConstraintTorqueY=off  SenseConstraintTorqueZ=off  SenseTotalForce=off  SenseTotalForceX=off  SenseTotalForceY=off  SenseTotalForceZ=off  SenseTotalTorque=off  SenseTotalTorqueX=off  SenseTotalTorqueY=off  SenseTotalTorqueZ=off  CompositeWrenchDir=FollowerOnBase  CompositeWrenchFrame=BaseFrame  EquilibriumPosition=0  EquilibriumPositionUnits=rad  SpringStiffness=0  SpringStiffnessUnits=N*m/rad  DampingCoefficient=0  DampingCoefficientUnits=N*m/(rad/s)  TorqueActuationMode=ComputedTorque  MotionActuationMode=InputMotion  SensePosition=off  SenseVelocity=off  SenseAcceleration=off  SenseTorqueForce=off  PositionTargetSpecify=on  PositionTargetPriority=Low  PositionTargetValue=smiData.RevoluteJoint(8).Rz.Pos  PositionTargetValueUnits=deg  VelocityTargetSpecify=off  VelocityTargetPriority=High  VelocityTargetValue=0  VelocityTargetValueUnits=deg/s
  Demux : Demux  Outputs=6
  Hip_joint : sm_lib/Joints/Revolute Joint  SenseConstraintForce=off  SenseConstraintForceX=off  SenseConstraintForceY=off  SenseConstraintForceZ=off  SenseConstraintTorque=off  SenseConstraintTorqueX=off  SenseConstraintTorqueY=off  SenseConstraintTorqueZ=off  SenseTotalForce=off  SenseTotalForceX=off  SenseTotalForceY=off  SenseTotalForceZ=off  SenseTotalTorque=off  SenseTotalTorqueX=off  SenseTotalTorqueY=off  SenseTotalTorqueZ=off  CompositeWrenchDir=FollowerOnBase  CompositeWrenchFrame=BaseFrame  EquilibriumPosition=0  EquilibriumPositionUnits=rad  SpringStiffness=0  SpringStiffnessUnits=N*m/rad  DampingCoefficient=0  DampingCoefficientUnits=N*m/(rad/s)  TorqueActuationMode=ComputedTorque  MotionActuationMode=InputMotion  SensePosition=off  SenseVelocity=off  SenseAcceleration=off  SenseTorqueForce=off  PositionTargetSpecify=on  PositionTargetPriority=Low  PositionTargetValue=smiData.RevoluteJoint(2).Rz.Pos  PositionTargetValueUnits=deg  VelocityTargetSpecify=off  VelocityTargetPriority=High  VelocityTargetValue=0  VelocityTargetValueUnits=deg/s
  Knee_Joint : sm_lib/Joints/Revolute Joint  SenseConstraintForce=off  SenseConstraintForceX=off  SenseConstraintForceY=off  SenseConstraintForceZ=off  SenseConstraintTorque=off  SenseConstraintTorqueX=off  SenseConstraintTorqueY=off  SenseConstraintTorqueZ=off  SenseTotalForce=off  SenseTotalForceX=off  SenseTotalForceY=off  SenseTotalForceZ=off  SenseTotalTorque=off  SenseTotalTorqueX=off  SenseTotalTorqueY=off  SenseTotalTorqueZ=off  CompositeWrenchDir=FollowerOnBase  CompositeWrenchFrame=BaseFrame  EquilibriumPosition=0  EquilibriumPositionUnits=rad  SpringStiffness=0  SpringStiffnessUnits=N*m/rad  DampingCoefficient=0  DampingCoefficientUnits=N*m/(rad/s)  TorqueActuationMode=ComputedTorque  MotionActuationMode=InputMotion  SensePosition=off  SenseVelocity=off  SenseAcceleration=off  SenseTorqueForce=off  PositionTargetSpecify=on  PositionTargetPriority=Low  PositionTargetValue=smiData.RevoluteJoint(1).Rz.Pos  PositionTargetValueUnits=deg  VelocityTargetSpecify=off  VelocityTargetPriority=High  VelocityTargetValue=0  VelocityTargetValueUnits=deg/s
  ReferenceFrame : sm_lib/Frames and Transforms/Reference Frame
  Rotation_joint : sm_lib/Joints/Revolute Joint  SenseConstraintForce=off  SenseConstraintForceX=off  SenseConstraintForceY=off  SenseConstraintForceZ=off  SenseConstraintTorque=off  SenseConstraintTorqueX=off  SenseConstraintTorqueY=off  SenseConstraintTorqueZ=off  SenseTotalForce=off  SenseTotalForceX=off  SenseTotalForceY=off  SenseTotalForceZ=off  SenseTotalTorque=off  SenseTotalTorqueX=off  SenseTotalTorqueY=off  SenseTotalTorqueZ=off  CompositeWrenchDir=FollowerOnBase  CompositeWrenchFrame=BaseFrame  EquilibriumPosition=0  EquilibriumPositionUnits=rad  SpringStiffness=0  SpringStiffnessUnits=N*m/rad  DampingCoefficient=0  DampingCoefficientUnits=N*m/(rad/s)  TorqueActuationMode=ComputedTorque  MotionActuationMode=InputMotion  SensePosition=off  SenseVelocity=off  SenseAcceleration=off  SenseTorqueForce=off  PositionTargetSpecify=on  PositionTargetPriority=Low  PositionTargetValue=smiData.RevoluteJoint(10).Rz.Pos  PositionTargetValueUnits=deg  VelocityTargetSpecify=off  VelocityTargetPriority=High  VelocityTargetValue=0  VelocityTargetValueUnits=deg/s
  Simulink-PS Converter{,1..5} (6 alike) : nesl_utility/Simulink-PS Converter  PhysicalDomain=network_engine_domain  SubClassName=ps_input  LeftPortType=input  RightPortType=output  PseudoPeriodic=off  Frequencies=[]  NoiseDistribution=none  NoiseParameters=[]  Unit=rad  AffineConversion=off  FilteringAndDerivatives=filter  SimscapeFilterOrder=2  InputFilterTimeConstant=motion_time_constant  UdotUserProvided=1
  Solid : sm_lib/Body Elements/Solid  InertiaType=Custom  Mass=smiData.Solid(9).mass  MassUnits=kg  CenterOfMass=smiData.Solid(9).CoM  CenterOfMassUnits=mm  MomentsOfInertia=smiData.Solid(9).MoI  MomentsOfInertiaUnits=kg*mm^2  ProductsOfInertia=smiData.Solid(9).PoI  ProductsOfInertiaUnits=kg*mm^2  DensityBased=on  Density=1000  DensityUnits=kg/m^3  DoExposeReferenceFrame=on  SerializedFrames=<Frames/>  GraphicType=FromGeometry  MarkerShape=Sphere  MarkerSize=10  GraphicVisPropType=SimpleVisualProperties  GraphicDiffuseColor=smiData.Solid(9).color  GraphicSpecularColor=[0.5 0.5 0.5 1.0]  GraphicAmbientColor=[0.15 0.15 0.15 1.0]  GraphicEmissiveColor=[0.0 0.0 0.0 1.0]  GraphicShininess=75  GraphicOpacity=smiData.Solid(9).opacity  GeometryShape=FromFile  RectangleSize=[1 1]  RectangleSizeUnits=m  BrickDimensions=[1 1 1]  BrickDimensionUnits=m  CylinderRadius=1  CylinderRadiusUnits=m  CylinderLength=1  CylinderLengthUnits=m  SphereRadius=1  SphereRadiusUnits=m  EllipsoidRadii=[1 1 1]  EllipsoidRadiiUnits=m  ExtrusionCrossSection=[1 1; -1 1; -1 -1; 1 -1]  ExtrusionCrossSectionUnits=m  ExtrusionLength=1  ExtrusionLengthUnits=m  PolygonNumSides=3  PolygonOuterRadius=1  PolygonOuterRadiusUnits=m  ExtGeomFileType=STEP  ExtGeomFileName=right_ankle_twist_part_Default_sldprt.STEP  ExtGeomFileUnits=m  RevolutionCrossSection=[1 1; 1 -1; 2 -1; 2 1]  RevolutionCrossSectionUnits=m  RevolutionExtent=Full  RevolutionAngle=180  RevolutionAngleUnits=deg
  Transform : sm_lib/Frames and Transforms/Rigid Transform  TranslationMethod=Cartesian  TranslationStandardOffset=0  TranslationLengthUnit=mm  TranslationStandardAxis=+Z  TranslationCartesianOffset=smiData.RigidTransform(16).translation  TranslationROffset=0  TranslationROffsetUnits=m  TranslationZOffset=0  TranslationZOffsetUnits=m  TranslationThetaOffset=0  TranslationThetaOffsetUnits=deg  RotationMethod=ArbitraryAxis  RotationAngleUnits=rad  RotationStandardAxis=+Z  RotationAngle=smiData.RigidTransform(16).angle  RotationArbitraryAxis=smiData.RigidTransform(16).axis  FollAlignAxisA=+X  BaseAlignAxisA=+Y  FollAlignAxisB=+Y  BaseAlignAxisB=+Z  RotationSequenceAxes=FollowerAxes  RotationSequence=XYX  RotationSequenceAngles=[0 0 0]  RotationSequenceAnglesUnits=deg  RotationMatrix=[1 0 0; 0 1 0; 0 0 1]
  right_abduction_RIGID : Subsystem
  right_ankle_RIGID : Subsystem
  right_flextion_RIGID : Subsystem
  right_knee_RIGID : Subsystem
  right_rotation_RIGID : Subsystem
  H : PMIOPort  Port=1  Side=Left
  wires:
  Demux/3 -> Simulink-PS Converter/1
  Demux/4 -> Simulink-PS Converter1/1
  Demux/5 -> Simulink-PS Converter5/1
  Demux/6 -> Simulink-PS Converter4/1
  Demux/2 -> Simulink-PS Converter2/1
  Demux/1 -> Simulink-PS Converter3/1
  qRef/1 -> Demux/1
  connections:
  Knee_Joint/RConn1 -- right_knee_RIGID/RConn1
  H/RConn1 -- Rotation_joint/LConn1
  Ankle_Twist_Joint/LConn1 -- right_ankle_RIGID/LConn1
  Knee_Joint/LConn1 -- right_flextion_RIGID/RConn1
  Abduction_joint/RConn1 -- right_rotation_RIGID/LConn1
  Ankle_Twist_Joint/RConn1 -- Transform/RConn1
  Rotation_joint/RConn1 -- right_rotation_RIGID/RConn1
  Ankle_Joint/LConn1 -- right_ankle_RIGID/RConn1
  Ankle_Joint/RConn1 -- right_knee_RIGID/LConn1
  Abduction_joint/LConn1 -- right_abduction_RIGID/RConn1
  Hip_joint/LConn1 -- right_abduction_RIGID/LConn1
  Hip_joint/RConn1 -- right_flextion_RIGID/LConn1
  ReferenceFrame/RConn1 -- Solid/RConn1 -- Transform/LConn1
  Rotation_joint/LConn2 -- Simulink-PS Converter4/RConn1
  Simulink-PS Converter5/RConn1 -- Abduction_joint/LConn2
  Knee_Joint/LConn2 -- Simulink-PS Converter/RConn1
  Simulink-PS Converter1/RConn1 -- Hip_joint/LConn2
  Simulink-PS Converter2/RConn1 -- Ankle_Joint/LConn2
  Ankle_Twist_Joint/LConn2 -- Simulink-PS Converter3/RConn1

== system Robot_leg_1/Robot/Left_leg/left_abduction_RIGID ==
  ReferenceFrame : sm_lib/Frames and Transforms/Reference Frame
  Solid : sm_lib/Body Elements/Solid  InertiaType=Custom  Mass=smiData.Solid(4).mass  MassUnits=kg  CenterOfMass=smiData.Solid(4).CoM  CenterOfMassUnits=mm  MomentsOfInertia=smiData.Solid(4).MoI  MomentsOfInertiaUnits=kg*mm^2  ProductsOfInertia=smiData.Solid(4).PoI  ProductsOfInertiaUnits=kg*mm^2  DensityBased=on  Density=1000  DensityUnits=kg/m^3  DoExposeReferenceFrame=on  SerializedFrames=<Frames/>  GraphicType=FromGeometry  MarkerShape=Sphere  MarkerSize=10  GraphicVisPropType=SimpleVisualProperties  GraphicDiffuseColor=smiData.Solid(4).color  GraphicSpecularColor=[0.5 0.5 0.5 1.0]  GraphicAmbientColor=[0.15 0.15 0.15 1.0]  GraphicEmissiveColor=[0.0 0.0 0.0 1.0]  GraphicShininess=75  GraphicOpacity=smiData.Solid(4).opacity  GeometryShape=FromFile  RectangleSize=[1 1]  RectangleSizeUnits=m  BrickDimensions=[1 1 1]  BrickDimensionUnits=m  CylinderRadius=1  CylinderRadiusUnits=m  CylinderLength=1  CylinderLengthUnits=m  SphereRadius=1  SphereRadiusUnits=m  EllipsoidRadii=[1 1 1]  EllipsoidRadiiUnits=m  ExtrusionCrossSection=[1 1; -1 1; -1 -1; 1 -1]  ExtrusionCrossSectionUnits=m  ExtrusionLength=1  ExtrusionLengthUnits=m  PolygonNumSides=3  PolygonOuterRadius=1  PolygonOuterRadiusUnits=m  ExtGeomFileType=STEP  ExtGeomFileName=left_abduction_part_Default_sldprt.STEP  ExtGeomFileUnits=m  RevolutionCrossSection=[1 1; 1 -1; 2 -1; 2 1]  RevolutionCrossSectionUnits=m  RevolutionExtent=Full  RevolutionAngle=180  RevolutionAngleUnits=deg
  Transform : sm_lib/Frames and Transforms/Rigid Transform  TranslationMethod=Cartesian  TranslationStandardOffset=0  TranslationLengthUnit=mm  TranslationStandardAxis=+Z  TranslationCartesianOffset=smiData.RigidTransform(7).translation  TranslationROffset=0  TranslationROffsetUnits=m  TranslationZOffset=0  TranslationZOffsetUnits=m  TranslationThetaOffset=0  TranslationThetaOffsetUnits=deg  RotationMethod=ArbitraryAxis  RotationAngleUnits=rad  RotationStandardAxis=+Z  RotationAngle=smiData.RigidTransform(7).angle  RotationArbitraryAxis=smiData.RigidTransform(7).axis  FollAlignAxisA=+X  BaseAlignAxisA=+Y  FollAlignAxisB=+Y  BaseAlignAxisB=+Z  RotationSequenceAxes=FollowerAxes  RotationSequence=XYX  RotationSequenceAngles=[0 0 0]  RotationSequenceAnglesUnits=deg  RotationMatrix=[1 0 0; 0 1 0; 0 0 1]
  Transform1 : sm_lib/Frames and Transforms/Rigid Transform  TranslationMethod=Cartesian  TranslationStandardOffset=0  TranslationLengthUnit=mm  TranslationStandardAxis=+Z  TranslationCartesianOffset=smiData.RigidTransform(25).translation  TranslationROffset=0  TranslationROffsetUnits=m  TranslationZOffset=0  TranslationZOffsetUnits=m  TranslationThetaOffset=0  TranslationThetaOffsetUnits=deg  RotationMethod=ArbitraryAxis  RotationAngleUnits=rad  RotationStandardAxis=+Z  RotationAngle=smiData.RigidTransform(25).angle  RotationArbitraryAxis=smiData.RigidTransform(25).axis  FollAlignAxisA=+X  BaseAlignAxisA=+Y  FollAlignAxisB=+Y  BaseAlignAxisB=+Z  RotationSequenceAxes=FollowerAxes  RotationSequence=XYX  RotationSequenceAngles=[0 0 0]  RotationSequenceAnglesUnits=deg  RotationMatrix=[1 0 0; 0 1 0; 0 0 1]
  F1 : PMIOPort  Port=1  Side=Right
  F : PMIOPort  Port=2  Side=Left
  connections:
  Solid/RConn1 -- ReferenceFrame/RConn1 -- Transform/LConn1 -- Transform1/LConn1
  Transform/RConn1 -- F/RConn1
  Transform1/RConn1 -- F1/RConn1

== system Robot_leg_1/Robot/Left_leg/left_ankle_RIGID ==
  ReferenceFrame : sm_lib/Frames and Transforms/Reference Frame
  Solid : sm_lib/Body Elements/Solid  InertiaType=Custom  Mass=smiData.Solid(7).mass  MassUnits=kg  CenterOfMass=smiData.Solid(7).CoM  CenterOfMassUnits=mm  MomentsOfInertia=smiData.Solid(7).MoI  MomentsOfInertiaUnits=kg*mm^2  ProductsOfInertia=smiData.Solid(7).PoI  ProductsOfInertiaUnits=kg*mm^2  DensityBased=on  Density=1000  DensityUnits=kg/m^3  DoExposeReferenceFrame=on  SerializedFrames=<Frames/>  GraphicType=FromGeometry  MarkerShape=Sphere  MarkerSize=10  GraphicVisPropType=SimpleVisualProperties  GraphicDiffuseColor=smiData.Solid(7).color  GraphicSpecularColor=[0.5 0.5 0.5 1.0]  GraphicAmbientColor=[0.15 0.15 0.15 1.0]  GraphicEmissiveColor=[0.0 0.0 0.0 1.0]  GraphicShininess=75  GraphicOpacity=smiData.Solid(7).opacity  GeometryShape=FromFile  RectangleSize=[1 1]  RectangleSizeUnits=m  BrickDimensions=[1 1 1]  BrickDimensionUnits=m  CylinderRadius=1  CylinderRadiusUnits=m  CylinderLength=1  CylinderLengthUnits=m  SphereRadius=1  SphereRadiusUnits=m  EllipsoidRadii=[1 1 1]  EllipsoidRadiiUnits=m  ExtrusionCrossSection=[1 1; -1 1; -1 -1; 1 -1]  ExtrusionCrossSectionUnits=m  ExtrusionLength=1  ExtrusionLengthUnits=m  PolygonNumSides=3  PolygonOuterRadius=1  PolygonOuterRadiusUnits=m  ExtGeomFileType=STEP  ExtGeomFileName=left_ankle_part_Default_sldprt.STEP  ExtGeomFileUnits=m  RevolutionCrossSection=[1 1; 1 -1; 2 -1; 2 1]  RevolutionCrossSectionUnits=m  RevolutionExtent=Full  RevolutionAngle=180  RevolutionAngleUnits=deg
  Transform : sm_lib/Frames and Transforms/Rigid Transform  TranslationMethod=Cartesian  TranslationStandardOffset=0  TranslationLengthUnit=mm  TranslationStandardAxis=+Z  TranslationCartesianOffset=smiData.RigidTransform(11).translation  TranslationROffset=0  TranslationROffsetUnits=m  TranslationZOffset=0  TranslationZOffsetUnits=m  TranslationThetaOffset=0  TranslationThetaOffsetUnits=deg  RotationMethod=ArbitraryAxis  RotationAngleUnits=rad  RotationStandardAxis=+Z  RotationAngle=smiData.RigidTransform(11).angle  RotationArbitraryAxis=smiData.RigidTransform(11).axis  FollAlignAxisA=+X  BaseAlignAxisA=+Y  FollAlignAxisB=+Y  BaseAlignAxisB=+Z  RotationSequenceAxes=FollowerAxes  RotationSequence=XYX  RotationSequenceAngles=[0 0 0]  RotationSequenceAnglesUnits=deg  RotationMatrix=[1 0 0; 0 1 0; 0 0 1]
  Transform1 : sm_lib/Frames and Transforms/Rigid Transform  TranslationMethod=Cartesian  TranslationStandardOffset=0  TranslationLengthUnit=mm  TranslationStandardAxis=+Z  TranslationCartesianOffset=smiData.RigidTransform(13).translation  TranslationROffset=0  TranslationROffsetUnits=m  TranslationZOffset=0  TranslationZOffsetUnits=m  TranslationThetaOffset=0  TranslationThetaOffsetUnits=deg  RotationMethod=ArbitraryAxis  RotationAngleUnits=rad  RotationStandardAxis=+Z  RotationAngle=smiData.RigidTransform(13).angle  RotationArbitraryAxis=smiData.RigidTransform(13).axis  FollAlignAxisA=+X  BaseAlignAxisA=+Y  FollAlignAxisB=+Y  BaseAlignAxisB=+Z  RotationSequenceAxes=FollowerAxes  RotationSequence=XYX  RotationSequenceAngles=[0 0 0]  RotationSequenceAnglesUnits=deg  RotationMatrix=[1 0 0; 0 1 0; 0 0 1]
  F1 : PMIOPort  Port=1  Side=Right
  F : PMIOPort  Port=2  Side=Left
  connections:
  Solid/RConn1 -- ReferenceFrame/RConn1 -- Transform/LConn1 -- Transform1/LConn1
  Transform/RConn1 -- F/RConn1
  Transform1/RConn1 -- F1/RConn1
